simulink model "SS_IEEE_9_bus_dynamic phasor"  (R2023b)
settings: Solver=VariableStepAuto  StartTime=0.0  StopTime=10.0  RelTol=1e-3
settings Model: Creator=dongyuli  LastModifiedBy=dongyuli

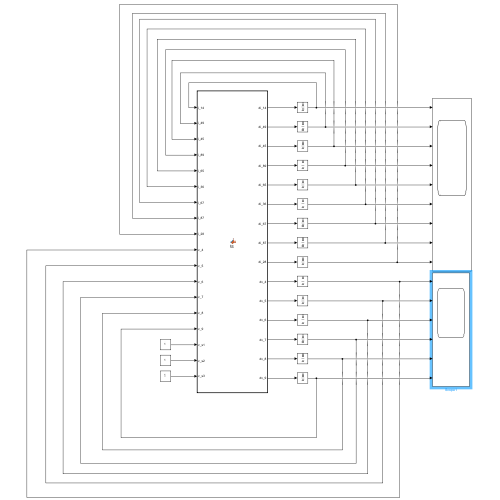
[thumbnail: Simulink's stored preview of the top-level diagram]
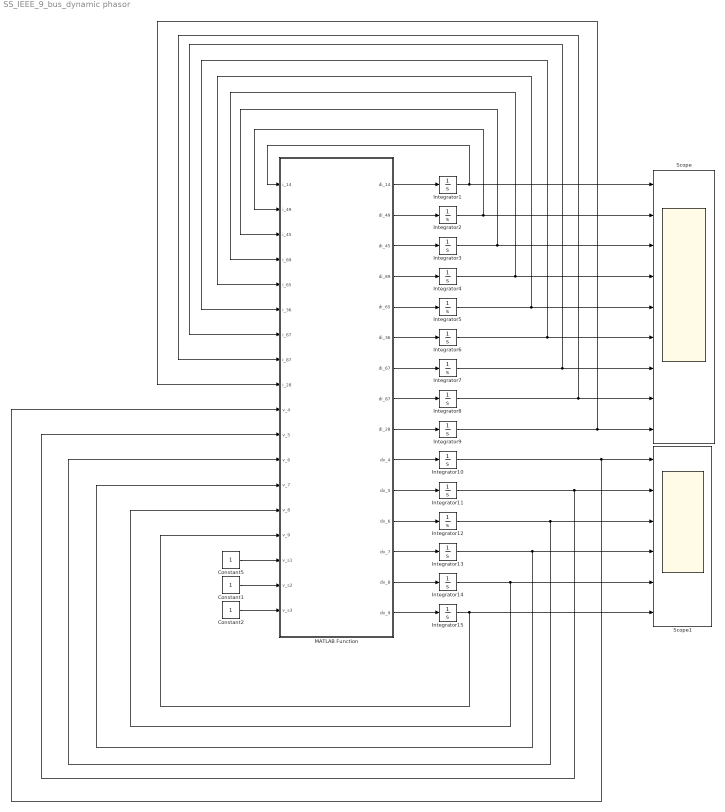
== system SS_IEEE_9_bus_dynamic phasor ==
  Constant1 : Constant
  Constant2 : Constant
  Constant5 : Constant
  Integrator{1..15} (15 alike) : Integrator
  MATLAB Function : MATLAB Function  TreatAsAtomicUnit=on
  Scope : Scope  NumInputPorts=9
  Scope1 : Scope  NumInputPorts=6
  wires:
  MATLAB Function/1(di_14) -> Integrator1/1
  MATLAB Function/2(di_49) -> Integrator2/1
  MATLAB Function/3(di_45) -> Integrator3/1
  MATLAB Function/4(di_89) -> Integrator4/1
  MATLAB Function/5(di_65) -> Integrator5/1
  MATLAB Function/6(di_36) -> Integrator6/1
  MATLAB Function/7(di_67) -> Integrator7/1
  MATLAB Function/8(di_87) -> Integrator8/1
  MATLAB Function/9(di_28) -> Integrator9/1
  MATLAB Function/10(dv_4) -> Integrator10/1
  MATLAB Function/11(dv_5) -> Integrator11/1
  MATLAB Function/12(dv_6) -> Integrator12/1
  MATLAB Function/13(dv_7) -> Integrator13/1
  MATLAB Function/14(dv_8) -> Integrator14/1
  MATLAB Function/15(dv_9) -> Integrator15/1
  Integrator1/1 -> Scope/1, MATLAB Function/1(i_14)
  Integrator2/1 -> Scope/2, MATLAB Function/2(i_49)
  Integrator3/1 -> Scope/3, MATLAB Function/3(i_45)
  Integrator4/1 -> Scope/4, MATLAB Function/4(i_89)
  Integrator5/1 -> Scope/5, MATLAB Function/5(i_65)
  Integrator6/1 -> Scope/6, MATLAB Function/6(i_36)
  Integrator7/1 -> Scope/7, MATLAB Function/7(i_67)
  Integrator8/1 -> Scope/8, MATLAB Function/8(i_87)
  Integrator9/1 -> Scope/9, MATLAB Function/9(i_28)
  Integrator10/1 -> Scope1/1, MATLAB Function/10(v_4)
  Integrator11/1 -> Scope1/2, MATLAB Function/11(v_5)
  Integrator12/1 -> Scope1/3, MATLAB Function/12(v_6)
  Integrator13/1 -> Scope1/4, MATLAB Function/13(v_7)
  Integrator14/1 -> Scope1/5, MATLAB Function/14(v_8)
  Integrator15/1 -> Scope1/6, MATLAB Function/15(v_9)
  Constant2/1 -> MATLAB Function/18(v_s3)
  Constant1/1 -> MATLAB Function/17(v_s2)
  Constant5/1 -> MATLAB Function/16(v_s1)

== matlab function SS_IEEE_9_bus_dynamic phasor/MATLAB Function ==
  data: i_14 input; di_14 output; di_49 output; di_45 output; di_89 output; di_65 output; di_36 output; di_67 output; di_87 output; di_28 output; dv_4 output; dv_5 output; dv_6 output; dv_7 output; dv_8 output; dv_9 output; i_49 input; i_45 input; i_89 input; i_65 input; i_36 input; i_67 input; i_87 input; i_28 input; v_4 input; v_5 input; v_6 input; v_7 input; v_8 input; v_9 input; v_s1 input; v_s2 input; v_s3 input
function [di_14, di_49, di_45, di_89, di_65, di_36, di_67, di_87, di_28, dv_4, dv_5, dv_6, dv_7, dv_8, dv_9] = fcn(i_14, i_49, i_45, i_89, i_65, i_36, i_67, i_87, i_28, v_4, v_5, v_6, v_7, v_8, v_9, v_s1, v_s2, v_s3)

f = 50;
w = 2*pi*f;

V_base = 345;
MVA_base = 100;
Z_base = (sqrt(3)*V_base^2)/MVA_base;

R_49 = 0.01*Z_base;
R_45 = 0.017*Z_base;
R_89 = 0.032*Z_base;
R_65 = 0.039*Z_base;
R_67 = 0.0119*Z_base;
R_87 = 0.0085*Z_base;

L_14 = 0.0576*Z_base/w;
L_49 = 0.085*Z_base/w;
L_45 = 0.092*Z_base/w;
L_89 = 0.161*Z_base/w;
L_65 = 0.170*Z_base/w;
L_36 = 0.0586*Z_base/w;
L_67 = 0.1008*Z_base/w;
L_87 = 0.072*Z_base/w;
L_28 = 0.0625*Z_base/w;

L_1 = 0.0608*Z_base/w;
L_2 = 0.1198*Z_base/w;
L_3 = 0.1813*Z_base/w;

C_4 = (0.079 + 0.088)*Z_base/w;
C_5 = (0.079 + 0.179)*Z_base/w;
C_6 = (0.179 + 0.1045)*Z_base/w;
C_7 = (0.1045 + 0.0745)*Z_base/w;
C_8 = (0.0745 + 0.153)*Z_base/w;
C_9 = (0.088 + 0.153)*Z_base/w;

X = [i_14, i_49, i_45, i_89, i_65, i_36, i_67, i_87, i_28, v_4, v_5, v_6, v_7, v_8, v_9]';

U = [v_s1, v_s2, v_s3]';

%A =[-R_14/L_14 0 0 0 0 0 0 0 0 1/L_14 0 0 -1/L_14 0 0 0 0 0;
%    0 -R_49/L_49 0 0 0 0 0 0 0 0 0 0 1/L_49 0 0 0 0 -1/L_49;
%    0 0 -R_45/L_45 0 0 0 0 0 0 0 0 0 1/L_45 -1/L_45 0 0 0 0;
%    0 0 0 -R_89/L_89 0 0 0 0 0 0 0 0 0 0 0 0 1/L_89 -1/L_89;
%    0 0 0 0 -R_65/L_65 0 0 0 0 0 0 0 0 -1/L_65 1/L_65 0 0 0;
%    0 0 0 0 0 -R_36/L_36 0 0 0 0 0 1/L_36 0 0 -1/L_36 0 0 0;
%    0 0 0 0 0 0 -R_67/L_67 0 0 0 0 0 0 0 1/L_67 -1/L_67 0 0;
%    0 0 0 0 0 0 0 -R_87/L_87 0 0 0 0 0 0 0 -1/L_87 1/L_87 0;
%    0 0 0 0 0 0 0 0 -R_28/L_28 0 1/L_28 0 0 0 0 0 -1/L_28 0;
%    -1/C_1 0 0 0 0 0 0 0 0 0 0 0 0 0 0 0 0 0;
%    0 0 0 0 0 0 0 0 -1/C_2 0 0 0 0 0 0 0 0 0;
%    0 0 0 0 0 -1/C_3 0 0 0 0 0 0 0 0 0 0 0 0;
%    1/C_4 -1/C_4 -1/C_4 0 0 0 0 0 0 0 0 0 0 0 0 0 0 0;
%    0 0 1/C_5 0 1/C_5 0 0 0 0 0 0 0 0 0 0 0 0 0;
%    0 0 0 0 -1/C_6 1/C_6 -1/C_6 0 0 0 0 0 0 0 0 0 0 0;
%    0 0 0 0 0 0 1/C_7 1/C_7 0 0 0 0 0 0 0 0 0 0;
%    0 0 0 -1/C_8 0 0 0 -1/C_8 1/C_8 0 0 0 0 0 0 0 0 0;
%    0 1/C_9 0 1/C_9 0 0 0 0 0 0 0 0 0 0 0 0 0 0];

A = [0 0 0 0 0 0 0 0 0 -1/(L_14+L_1) 0 0 0 0 0;
    0 -R_49/L_49 0 0 0 0 0 0 0 1/L_49 0 0 0 0 -1/L_49;
    0 0 -R_45/L_45 0 0 0 0 0 0 1/L_45 -1/L_45 0 0 0 0;
    0 0 0 -R_89/L_89 0 0 0 0 0 0 0 0 0 1/L_89 -1/L_89;
    0 0 0 0 -R_65/L_65 0 0 0 0 0 -1/L_65 1/L_65 0 0 0;
    0 0 0 0 0 0 0 0 0 0 0 -1/(L_36+L_3) 0 0 0;
    0 0 0 0 0 0 -R_67/L_67 0 0 0 0 1/L_67 -1/L_67 0 0;
    0 0 0 0 0 0 0 -R_87/L_87 0 0 0 0 0 -1/L_87 1/L_87;
    0 0 0 0 0 0 0 0 0 0 0 0 0 -1/(L_28+L_2) 0;
    1/C_4 -1/C_4 -1/C_4 0 0 0 0 0 0 0 0 0 0 0 0;
    0 0 1/C_5 0 1/C_5 0 0 0 0 0 0 0 0 0 0;
    0 0 0 0 -1/C_6 1/C_6 -1/C_6 0 0 0 0 0 0 0 0;
    0 0 0 0 0 0 1/C_7 1/C_7 0 0 0 0 0 0 0;
    0 0 0 0 -1/C_8 0 0 -1/C_8 1/C_8 0 0 0 0 0 0;
    0 1/C_9 0 1/C_9 0 0 0 0 0 0 0 0 0 0 0];

B =[1/(L_14+L_1) 0 0;
    0 0 0;
    0 0 0;
    0 0 0;
    0 0 0;
    0 0 1/(L_36+L_3);
    0 0 0;
    0 0 0;
    0 1/(L_28+L_2) 0;
    0 0 0;
    0 0 0;
    0 0 0;
    0 0 0;
    0 0 0;
    0 0 0];

dX = A*X + B*U;

di_14 = dX(1);
di_49 = dX(2);
di_45 = dX(3);
di_89 = dX(4);
di_65 = dX(5);
di_36 = dX(6);
di_67 = dX(7);
di_87 = dX(8);
di_28 = dX(9);

dv_4 = dX(10);
dv_5 = dX(11);
dv_6 = dX(12);
dv_7 = dX(13);
dv_8 = dX(14);
dv_9 = dX(15);

end
